simulink model "spaceshipWSOUT"  (Simulink 6.1)
settings: Solver=ode45  StartTime=0.0  StopTime=10.0  RelTol=1e-3
settings Model: LastModifiedBy=okawa
settings DebuggingCC: SolverPrmCheckMsg=warning

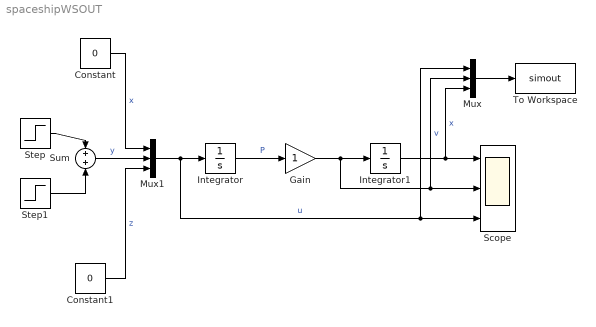
== system spaceshipWSOUT ==
  Constant : Constant  Value=0
  Constant1 : Constant  Value=0
  Gain : Gain
  Integrator : Integrator
  Integrator1 : Integrator
  Mux : Mux  Inputs=3
  Mux1 : Mux  Inputs=3
  Scope : Scope  NumInputPorts=3
      settings: YMin=-5~-5~-5  YMax=5~5~5
  Step : Step  SampleTime=0
  Step1 : Step  Time=2  After=-1  SampleTime=0
  Sum : Sum  Inputs=+|+
  To Workspace : ToWorkspace  VariableName=simout  SampleTime=-1  SaveFormat=Array
  wires:
  Constant/1 -> Mux1/1  "x"
  Constant1/1 -> Mux1/3  "z"
  Integrator1/1 -> Scope/1, Mux/3  "x"
  Sum/1 -> Mux1/2  "y"
  Step/1 -> Sum/1
  Step1/1 -> Sum/2
  Mux1/1 -> Integrator/1, Scope/3, Mux/1  "u"
  Integrator/1 -> Gain/1  "P"
  Gain/1 -> Integrator1/1, Scope/2, Mux/2  "v"
  Mux/1 -> To Workspace/1
